simulink model "questA_feedback_model"  (R2018a)
settings: Solver=VariableStepAuto  StartTime=0.0  StopTime=3  RelTol=1e-3
values from neighbouring files (symbols this model uses):
  A = [0 1 0 0; 20.6 0 0 0; 0 0 0 1; -.5 0 0 0]    [InvertedPendulum.m]
  B = [0; -1; 0; .5]    [InvertedPendulum.m]
  C = [1 0 0 0; 0 0 1 0]    [InvertedPendulum.m]
  K = place(A, B, p)    [InvertedPendulum.m]
  x0 = [-.2; -.06; .01; .3]    [InvertedPendulum.m]
settings Model: Creator=Administrator  LastModifiedBy=patsa

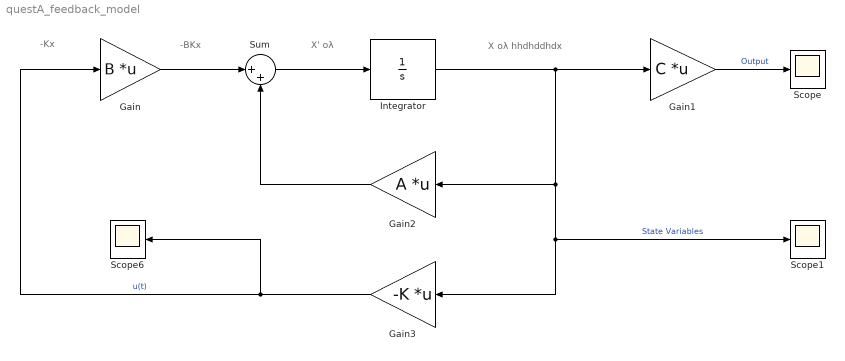
== system questA_feedback_model ==
  note: -Kx
  note: X ολ
      |
      | hhdhddhdx
  note: -BKx
  note: X' ολ
  Gain : Gain  Gain=B  Multiplication=Matrix(K*u)
  Gain1 : Gain  Gain=C  Multiplication=Matrix(K*u)
  Gain2 : Gain  Gain=A  Multiplication=Matrix(K*u)
  Gain3 : Gain  Gain=-K  Multiplication=Matrix(K*u)
  Integrator : Integrator  InitialCondition=x0
  Scope : Scope
  Scope1 : Scope
  Scope6 : Scope
  Sum : Sum  Inputs=|++
  wires:
  Sum/1 -> Integrator/1
  Integrator/1 -> Gain1/1, Scope1/1, Gain3/1, Gain2/1  "State Variables"
  Gain/1 -> Sum/1
  Gain1/1 -> Scope/1  "Output"
  Gain2/1 -> Sum/2
  Gain3/1 -> Gain/1, Scope6/1  "u(t)"
